simulink model "ev_supervisory_control"  (Simulink 8.1)
settings: Solver=ode3  StartTime=0  StopTime=10000  FixedStep=1  RelTol=1e-3
libraries: CampusEnergyModeling x4, simulink x1
settings Model: Creator=sfrank1  LastModifiedBy=sfrank1
settings DataIOCC: SignalLoggingSaveFormat=Dataset
settings OptimizationCC: ExpressionDepthLimit=128
settings DebuggingCC: FcnCallInpInsideContextMsg=EnableAllAsError
settings GRTTargetCC: CombineOutputUpdateFcns=on  GRTInterface=off

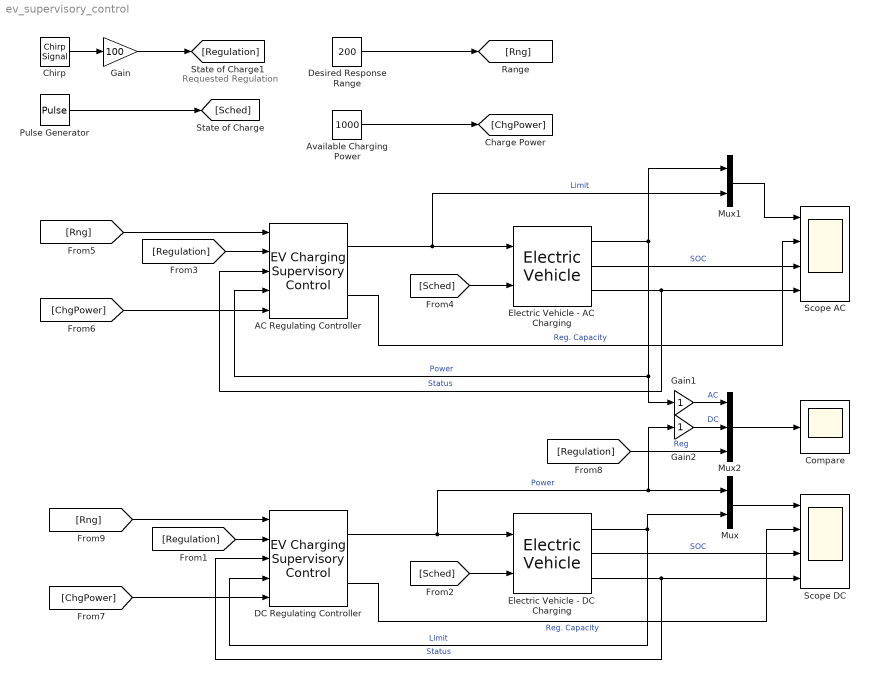
== system ev_supervisory_control ==
  note: Requested Regulation
  AC Regulating Controller : CampusEnergyModeling/Electric Vehicles/EV Charging Supervisory Control  ctype=AC  ramp=2  ldsettings=on  sweepint=300  sweepramp=0.5  thr=1.0
  Available Charging Power : Constant  Value=1000
  Chirp : simulink/Sources/Chirp Signal  f1=1/2000  T=10e3  f2=1/200
  Compare : Scope
      settings: ShowLegends=on  TimeRange=10000  YMin=-100  YMax=900  SaveName=ScopeData2
  DC Regulating Controller : CampusEnergyModeling/Electric Vehicles/EV Charging Supervisory Control  ctype=DC  ramp=2  ldsettings=off  sweepint=300  sweepramp=2  thr=1.0
  Desired Response Range : Constant  Value=200
  Electric Vehicle - AC Charging : CampusEnergyModeling/Electric Vehicles/Electric Vehicle  ctype=AC  rating=1000  chargerEff=0.96  profile=off  profileSOC=[0.00 0.10 0.20 0.80 0.99 1.00]  profileRate=[0.10 0.20 1.00 1.00 0.01 0.00]  capacity=1000  initSOC=0.1  battEff=0.98
  Electric Vehicle - DC Charging : CampusEnergyModeling/Electric Vehicles/Electric Vehicle  ctype=DC  rating=6240  chargerEff=0.96  profile=off  profileSOC=[0.00 0.10 0.20 0.80 0.99 1.00]  profileRate=[0.10 0.20 1.00 1.00 0.01 0.00]  capacity=1000  initSOC=0.1  battEff=0.98
  Gain : Gain  Gain=100
  Gain1 : Gain
  Gain2 : Gain
  Mux : Mux  Inputs=2
  Mux1 : Mux  Inputs=2
  Mux2 : Mux  Inputs=3
  Pulse Generator : DiscretePulseGenerator  PulseType=Time based  Period=10000  PulseWidth=80  PhaseDelay=1000
  Scope AC : Scope  NumInputPorts=4
      settings: ShowLegends=on  TimeRange=10000  YMin=0~0~0~-1  YMax=1000~200~1~0
  Scope DC : Scope  NumInputPorts=4
      settings: ShowLegends=on  TimeRange=10000  YMin=0~0~0~-1  YMax=1000~200~1~0
  wires:
  Electric Vehicle - DC Charging/1 -> DC Regulating Controller/4, Mux/2  "Limit"
  DC Regulating Controller/1 -> Electric Vehicle - DC Charging/1, Gain2/1, Mux/1  "Power"
  Pulse Generator/1 -> [Sched]
  [Sched] -> Electric Vehicle - DC Charging/2
  Chirp/1 -> Gain/1
  Gain/1 -> [Regulation]
  Electric Vehicle - DC Charging/2 -> Scope DC/3  "SOC"
  Electric Vehicle - DC Charging/3 -> DC Regulating Controller/3, Scope DC/4  "Status"
  DC Regulating Controller/2 -> Scope DC/2  "Reg. Capacity"
  Mux/1 -> Scope DC/1
  AC Regulating Controller/1 -> Mux1/2, Electric Vehicle - AC Charging/1  "Limit"
  [Sched] -> Electric Vehicle - AC Charging/2
  [Regulation] -> AC Regulating Controller/2
  Electric Vehicle - AC Charging/2 -> Scope AC/3  "SOC"
  Electric Vehicle - AC Charging/3 -> AC Regulating Controller/3, Scope AC/4  "Status"
  AC Regulating Controller/2 -> Scope AC/2  "Reg. Capacity"
  Mux1/1 -> Scope AC/1
  Electric Vehicle - AC Charging/1 -> Gain1/1, AC Regulating Controller/4, Mux1/1  "Power"
  Mux2/1 -> Compare/1
  Gain1/1 -> Mux2/1  "AC"
  Gain2/1 -> Mux2/2  "DC"
  Available Charging Power/1 -> [ChgPower]
  Desired Response Range/1 -> [Rng]
  [Rng] -> AC Regulating Controller/1
  [ChgPower] -> AC Regulating Controller/5
  [ChgPower] -> DC Regulating Controller/5
  [Regulation] -> Mux2/3  "Reg"
  [Rng] -> DC Regulating Controller/1
  [Regulation] -> DC Regulating Controller/2
